simulink library "isi_correlator_lib"  (Simulink 7.4)
settings: Solver=ode45  SolverMode=SingleTasking  StartTime=0.0  StopTime=10.0  RelTol=1e-3
undefined symbols (not defined in the file or in its folder): latency
libraries: xbsIndex_r4 x341, isi_correlator_lib x33, casper_library x27, xps_library x7
(part 2 of 3)

== system isi_correlator_lib/scale ==
  din : Inport  OutDataType=sfix(16)  OutScaling=2^0
  scale : Inport  Port=2  OutDataType=sfix(16)  OutScaling=2^0
  Assert0 : xbsIndex_r4/Assert  assert_type=on  type_source=Explicitly  arith_type=Unsigned  n_bits=2 * data_bit_width  bin_pt=0  assert_rate=on  rate_source=Explicitly  period=1  output_port=on  block_type=assert
      settings: block_version=11.4
  Assert1 : xbsIndex_r4/Assert  assert_type=on  type_source=Explicitly  arith_type=Unsigned  n_bits=coef_bit_width  bin_pt=0  assert_rate=on  rate_source=Explicitly  period=1  output_port=on  block_type=assert
      settings: block_version=11.4
  Logical : xbsIndex_r4/Logical  logical_function=OR  inputs=2  en=off  latency=0  precision=Full  arith_type=Unsigned  n_bits=8  bin_pt=2  align_bp=on  dbl_ovrd=off  block_type=logical
      settings: xl_area=[0, 0, 0, 0, 0, 0, 0]
  Mult_imag : xbsIndex_r4/Mult  precision=Full  arith_type="Signed  (2's comp)"  n_bits=16  bin_pt=14  quantization=Truncate  overflow=Wrap  en=off  latency=3  dbl_ovrd=off  use_behavioral_HDL=off  opt=Speed  use_embedded=on  optimum_pipeline=off  pipeline=on  use_rpm=on  placement_style=Triangular  block_type=mult
      settings: infoedit=Hardware notes: To use the internal pipeline stage of the dedicated multiplier you must select 'Pipeline for maximum performance'.  block_version=10.1.3
  Mult_real : xbsIndex_r4/Mult  precision=Full  arith_type="Signed  (2's comp)"  n_bits=16  bin_pt=14  quantization=Truncate  overflow=Wrap  en=off  latency=3  dbl_ovrd=off  use_behavioral_HDL=off  opt=Speed  use_embedded=on  optimum_pipeline=off  pipeline=on  use_rpm=on  placement_style=Triangular  block_type=mult
      settings: infoedit=Hardware notes: To use the internal pipeline stage of the dedicated multiplier you must select 'Pipeline for maximum performance'.  block_version=10.1.3
  c_to_ri : casper_library/Misc/c_to_ri  SystemSampleTime=-1  n_bits=data_bit_width  bin_pt=data_bit_width - 1
      settings: AttributesFormatString=_ r/i
  ri_to_c : casper_library/Misc/ri_to_c  SystemSampleTime=-1
  saturate_imag : isi_correlator_lib/saturate  SystemSampleTime=-1  data_bit_width=data_bit_width  dout_bit_width=dout_bit_width
  saturate_real : isi_correlator_lib/saturate  SystemSampleTime=-1  data_bit_width=data_bit_width  dout_bit_width=dout_bit_width
  dout : Outport  OutDataType=sfix(16)  OutScaling=2^0
  clip : Outport  Port=2  OutDataType=sfix(16)  OutScaling=2^0
  wires:
  Assert1/1 -> Mult_real/2, Mult_imag/2
  c_to_ri/2 -> Mult_imag/1
  Logical/1 -> clip/1
  scale/1 -> Assert1/1
  c_to_ri/1 -> Mult_real/1
  ri_to_c/1 -> dout/1
  Mult_real/1 -> saturate_real/1
  Mult_imag/1 -> saturate_imag/1
  saturate_real/1 -> ri_to_c/1
  saturate_imag/1 -> ri_to_c/2
  saturate_real/2 -> Logical/1
  saturate_imag/2 -> Logical/2
  din/1 -> Assert0/1
  Assert0/1 -> c_to_ri/1

== system isi_correlator_lib/simple_bram_vacc ==
  new_acc : Inport  OutDataType=sfix(16)  OutScaling=2^0
  din : Inport  Port=2  OutDataType=sfix(16)  OutScaling=2^0
  Adder : xbsIndex_r4/AddSub  mode=Addition  use_carryin=off  use_carryout=off  en=off  latency=2  precision=User Defined  arith_type="Signed  (2's comp)"  n_bits=n_bits  bin_pt=bin_pt  quantization=Truncate  overflow=Wrap  dbl_ovrd=off  use_behavioral_HDL=off  hw_selection=Fabric  pipelined=on  use_rpm=on  block_type=addsub
      settings: xl_area=[0, 0, 0, 0, 0, 0, 0]  block_version=10.1.3
  Constant : xbsIndex_r4/Constant  arith_type=Signed (2's comp)  const=0  n_bits=n_bits  bin_pt=bin_pt  explicit_period=on  period=1  equ=P=C  opselect=C  inp2=PCIN>>17  opr=+  inp1=P  carry=CIN  dbl_ovrd=off  block_type=constant
  Mux : xbsIndex_r4/Mux  inputs=2  en=off  latency=0  precision=Full  arith_type="Signed  (2's comp)"  n_bits=8  bin_pt=2  quantization=Truncate  overflow=Wrap  dbl_ovrd=off  block_type=mux
      settings: xl_area=[0, 0, 0, 0, 0, 0, 0]
  delay_bram : Subsystem  mask(delay_bram){DelayLen=vec_len - 2, bram_latency=2}
      mask prompts: DelayLen "Delay By:"; bram_latency "BRAM Latency"
      mask help: A delay block that uses BRAM for its storage.
      mask init:
      | if (DelayLen <= bram_latency)
      | 	error('delay value must be greater than BRAM Latency');
      | end
      | BitWidth = max(ceil(log2(DelayLen)), 2);
      mask Help: eval('xlWeb(''http://casper.berkeley.edu/wiki/Delay_bram'')')
  pulse_ext : Subsystem  mask(pulse_ext){pulse_len=vec_len}
      mask prompts: pulse_len "Length of Pulse"
      mask help:
      | Extends a boolean signal to be high for the specified number of clocks after
      | the last high input.
      mask init:
      | bits = ceil(log2(pulse_len+1));
      mask Help: eval('xlWeb(''http://casper.berkeley.edu/wiki/Pulse_ext'')')
  dout : Outport  OutDataType=sfix(16)  OutScaling=2^0
  valid : Outport  Port=2  OutDataType=sfix(16)  OutScaling=2^0
  wires:
  Adder/1 -> delay_bram/1(In1)
  delay_bram/1(Out1) -> dout/1, Mux/2
  new_acc/1 -> pulse_ext/1(in)
  din/1 -> Adder/1
  pulse_ext/1(out) -> valid/1, Mux/1
  Mux/1 -> Adder/2
  Constant/1 -> Mux/3

== system isi_correlator_lib/sync_gen ==
  rst : Inport  OutDataType=sfix(16)  OutScaling=2^0
  AddSub : xbsIndex_r4/AddSub  mode=Subtraction  use_carryin=off  use_carryout=off  en=off  latency=2  precision=Full  arith_type=Unsigned  n_bits=16  bin_pt=14  quantization=Truncate  overflow=Wrap  dbl_ovrd=off  use_behavioral_HDL=off  hw_selection=Fabric  pipelined=off  use_rpm=on  block_type=addsub
      settings: block_version=10.1.3
  Delay : xbsIndex_r4/Delay  en=off  latency=3  dbl_ovrd=off  reg_retiming=on  block_type=delay
      settings: block_version=11.3
  Logical1 : xbsIndex_r4/Logical  logical_function=OR  inputs=2  en=off  latency=0  precision=Full  arith_type=Unsigned  n_bits=16  bin_pt=0  align_bp=on  dbl_ovrd=off  block_type=logical
  Relational : xbsIndex_r4/Relational  mode=a>=b  en=off  latency=1  dbl_ovrd=off  block_type=relational
      settings: block_version=10.1.3
  counter : xbsIndex_r4/Counter  cnt_type=Free Running  cnt_to=Inf  operation=Up  start_count=0  cnt_by_val=1  arith_type=Unsigned  n_bits=32  bin_pt=0  load_pin=off  rst=on  en=off  explicit_period=on  period=1  dbl_ovrd=off  use_behavioral_HDL=off  implementation=Fabric  use_rpm=off  block_type=counter
  default_period : Constant  Value=1024  OutDataType=sfix(16)  OutScaling=2^0  SampleTime=1
  period : xps_library/software register  Tag=xps:sw_reg  SystemSampleTime=-1  io_dir=From Processor  arith_type=Unsigned  bitwidth=32  bin_pt=0  sample_period=1  gw_name=isi_correlator_lib_sync_gen_period_user_data_out
  period_offset : xbsIndex_r4/Constant  arith_type=Unsigned  const=3  n_bits=32  bin_pt=0  explicit_period=on  period=1  equ=P=C  opselect=C  inp2=PCIN>>17  opr=+  inp1=P  carry=CIN  dbl_ovrd=off  block_type=constant
      settings: block_version=10.1.1
  posedge : casper_library/Misc/posedge  Tag=Rising Edge Detector  SystemSampleTime=-1
  sync : Outport  OutDataType=sfix(16)  OutScaling=2^0
  wires:
  rst/1 -> Logical1/2
  Relational/1 -> Logical1/1
  posedge/1 -> sync/1
  Logical1/1 -> counter/1, posedge/1
  counter/1 -> Relational/1
  AddSub/1 -> Relational/2
  period_offset/1 -> AddSub/2
  default_period/1 -> period/1
  period/1 -> Delay/1
  Delay/1 -> AddSub/1

== system isi_correlator_lib/synced_cntr ==
  sync : Inport
  Constant : xbsIndex_r4/Constant  arith_type=Unsigned  const=0  n_bits=nextpow2(period)  bin_pt=0  explicit_period=on  period=1  equ=P=C  opselect=C  inp2=PCIN>>17  opr=+  inp1=P  carry=CIN  dbl_ovrd=off  block_type=constant
      settings: block_version=11.4
  Constant3 : xbsIndex_r4/Constant  arith_type=Unsigned  const=period - 1  n_bits=nextpow2(period)  bin_pt=0  explicit_period=on  period=1  equ=P=C  opselect=C  inp2=PCIN>>17  opr=+  inp1=P  carry=CIN  dbl_ovrd=off  block_type=constant
      settings: block_version=11.4
  Counter : xbsIndex_r4/Counter  cnt_type=Free Running  cnt_to=Inf  operation=Up  start_count=0  cnt_by_val=1  arith_type=Unsigned  n_bits=nextpow2(period)  bin_pt=0  load_pin=on  rst=off  en=off  explicit_period=on  period=1  dbl_ovrd=off  use_behavioral_HDL=off  implementation=Fabric  use_rpm=off  block_type=counter
  Logical2 : xbsIndex_r4/Logical  logical_function=OR  inputs=2  en=off  latency=0  precision=Full  arith_type=Unsigned  n_bits=16  bin_pt=0  align_bp=on  dbl_ovrd=off  block_type=logical
      settings: block_version=11.3
  Relational2 : xbsIndex_r4/Relational  mode=a=b  en=off  latency=0  dbl_ovrd=off  block_type=relational
  cnt : Outport
  wires:
  Constant/1 -> Counter/2
  sync/1 -> Logical2/2
  Logical2/1 -> Counter/1
  Counter/1 -> cnt/1, Relational2/2
  Constant3/1 -> Relational2/1
  Relational2/1 -> Logical2/1

== system isi_correlator_lib/trig_cntr ==
  trig : Inport
  Counter : xbsIndex_r4/Counter  cnt_type=Free Running  cnt_to=Inf  operation=Up  start_count=0  cnt_by_val=1  arith_type=Unsigned  n_bits=bitwidth + 1  bin_pt=0  load_pin=off  rst=on  en=on  explicit_period=on  period=1  dbl_ovrd=off  use_behavioral_HDL=off  implementation=Fabric  use_rpm=off  block_type=counter
  Inverter : xbsIndex_r4/Inverter  en=off  latency=0  dbl_ovrd=off  block_type=inv
      settings: block_version=11.3
  Inverter1 : xbsIndex_r4/Inverter  en=off  latency=0  dbl_ovrd=off  block_type=inv
      settings: block_version=11.3
  Logical : xbsIndex_r4/Logical  logical_function=AND  inputs=2  en=off  latency=latency  precision=Full  arith_type=Unsigned  n_bits=16  bin_pt=0  align_bp=on  dbl_ovrd=off  block_type=logical
      settings: block_version=11.3
  address : xbsIndex_r4/Slice  nbits=bitwidth  boolean_output=off  mode=Lower Bit Location + Width  bit1=0  base1=MSB of Input  bit0=0  base0=LSB of Input  dbl_ovrd=off  block_type=slice
      settings: block_version=10.1.1
  cntr_delay0 : xbsIndex_r4/Delay  en=off  latency=latency  dbl_ovrd=off  reg_retiming=on  block_type=delay
      settings: block_version=11.3
  overflow : xbsIndex_r4/Slice  nbits=1  boolean_output=on  mode=Upper Bit Location + Width  bit1=0  base1=MSB of Input  bit0=0  base0=LSB of Input  dbl_ovrd=off  block_type=slice
      settings: block_version=10.1.1
  addr : Outport
  we : Outport  Port=2
  wires:
  Counter/1 -> overflow/1, address/1
  trig/1 -> Counter/1, Inverter1/1
  address/1 -> cntr_delay0/1
  overflow/1 -> Inverter/1
  Inverter/1 -> Counter/2, Logical/1
  Inverter1/1 -> Logical/2
  Logical/1 -> we/1
  cntr_delay0/1 -> addr/1

== system isi_correlator_lib/tvg ==
  sync : Inport
  Constant : xbsIndex_r4/Constant  arith_type=Unsigned  const=0  n_bits=32  bin_pt=0  explicit_period=on  period=1  equ=P=C  opselect=C  inp2=PCIN>>17  opr=+  inp1=P  carry=CIN  dbl_ovrd=off  block_type=constant
  Constant1 : xbsIndex_r4/Constant  arith_type=Boolean  const=0  n_bits=32  bin_pt=0  explicit_period=on  period=1  equ=P=C  opselect=C  inp2=PCIN>>17  opr=+  inp1=P  carry=CIN  dbl_ovrd=off  block_type=constant
  bram : xps_library/Shared BRAM  Tag=xps:bram  SystemSampleTime=-1  arith_type="Signed  (2's comp)"  addr_width=nextpow2(length)  data_width=32  data_bin_pt=0  init_vals=[1:2^nextpow2(length)]  sample_rate=1
  delay3 : xbsIndex_r4/Delay  en=off  latency=1  dbl_ovrd=off  reg_retiming=off  block_type=delay
  synced_cntr : isi_correlator_lib/synced_cntr  SystemSampleTime=-1  period=length
  sync_out : Outport
  dout : Outport  Port=2
  wires:
  delay3/1 -> sync_out/1
  bram/1 -> dout/1
  synced_cntr/1 -> bram/1
  sync/1 -> delay3/1, synced_cntr/1
  Constant/1 -> bram/2
  Constant1/1 -> bram/3

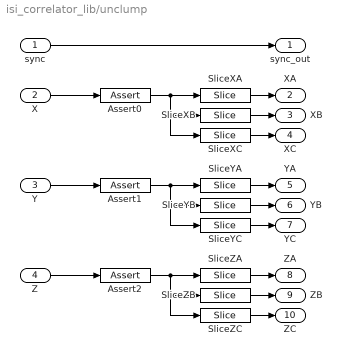
== system isi_correlator_lib/unclump ==
  sync : Inport
  X : Inport  Port=2
  Y : Inport  Port=3
  Z : Inport  Port=4
  Assert0 : xbsIndex_r4/Assert  assert_type=on  type_source=Explicitly  arith_type=Unsigned  n_bits=24  bin_pt=0  assert_rate=on  rate_source=Explicitly  period=1  output_port=on  block_type=assert
      settings: block_version=11.4
  Assert1 : xbsIndex_r4/Assert  assert_type=on  type_source=Explicitly  arith_type=Unsigned  n_bits=24  bin_pt=0  assert_rate=on  rate_source=Explicitly  period=1  output_port=on  block_type=assert
      settings: block_version=11.4
  Assert2 : xbsIndex_r4/Assert  assert_type=on  type_source=Explicitly  arith_type=Unsigned  n_bits=24  bin_pt=0  assert_rate=on  rate_source=Explicitly  period=1  output_port=on  block_type=assert
      settings: block_version=11.4
  SliceXA : xbsIndex_r4/Slice  nbits=8  boolean_output=off  mode=Lower Bit Location + Width  bit1=0  base1=MSB of Input  bit0=16  base0=LSB of Input  dbl_ovrd=off  block_type=slice
      settings: block_version=10.1.1
  SliceXB : xbsIndex_r4/Slice  nbits=8  boolean_output=off  mode=Lower Bit Location + Width  bit1=0  base1=MSB of Input  bit0=8  base0=LSB of Input  dbl_ovrd=off  block_type=slice
      settings: block_version=10.1.1
  SliceXC : xbsIndex_r4/Slice  nbits=8  boolean_output=off  mode=Lower Bit Location + Width  bit1=0  base1=MSB of Input  bit0=0  base0=LSB of Input  dbl_ovrd=off  block_type=slice
      settings: block_version=10.1.1
  SliceYA : xbsIndex_r4/Slice  nbits=8  boolean_output=off  mode=Lower Bit Location + Width  bit1=0  base1=MSB of Input  bit0=16  base0=LSB of Input  dbl_ovrd=off  block_type=slice
      settings: block_version=10.1.1
  SliceYB : xbsIndex_r4/Slice  nbits=8  boolean_output=off  mode=Lower Bit Location + Width  bit1=0  base1=MSB of Input  bit0=8  base0=LSB of Input  dbl_ovrd=off  block_type=slice
      settings: block_version=10.1.1
  SliceYC : xbsIndex_r4/Slice  nbits=8  boolean_output=off  mode=Lower Bit Location + Width  bit1=0  base1=MSB of Input  bit0=0  base0=LSB of Input  dbl_ovrd=off  block_type=slice
      settings: block_version=10.1.1
  SliceZA : xbsIndex_r4/Slice  nbits=8  boolean_output=off  mode=Lower Bit Location + Width  bit1=0  base1=MSB of Input  bit0=16  base0=LSB of Input  dbl_ovrd=off  block_type=slice
      settings: block_version=10.1.1
  SliceZB : xbsIndex_r4/Slice  nbits=8  boolean_output=off  mode=Lower Bit Location + Width  bit1=0  base1=MSB of Input  bit0=8  base0=LSB of Input  dbl_ovrd=off  block_type=slice
      settings: block_version=10.1.1
  SliceZC : xbsIndex_r4/Slice  nbits=8  boolean_output=off  mode=Lower Bit Location + Width  bit1=0  base1=MSB of Input  bit0=0  base0=LSB of Input  dbl_ovrd=off  block_type=slice
      settings: block_version=10.1.1
  sync_out : Outport
  XA : Outport  Port=2
  XB : Outport  Port=3
  XC : Outport  Port=4
  YA : Outport  Port=5
  YB : Outport  Port=6
  YC : Outport  Port=7
  ZA : Outport  Port=8
  ZB : Outport  Port=9
  ZC : Outport  Port=10
  wires:
  SliceZC/1 -> ZC/1
  SliceZB/1 -> ZB/1
  SliceZA/1 -> ZA/1
  SliceYC/1 -> YC/1
  SliceYB/1 -> YB/1
  SliceYA/1 -> YA/1
  SliceXC/1 -> XC/1
  SliceXB/1 -> XB/1
  SliceXA/1 -> XA/1
  Assert2/1 -> SliceZB/1, SliceZC/1, SliceZA/1
  Assert1/1 -> SliceYB/1, SliceYC/1, SliceYA/1
  Assert0/1 -> SliceXB/1, SliceXC/1, SliceXA/1
  Z/1 -> Assert2/1
  Y/1 -> Assert1/1
  X/1 -> Assert0/1
  sync/1 -> sync_out/1

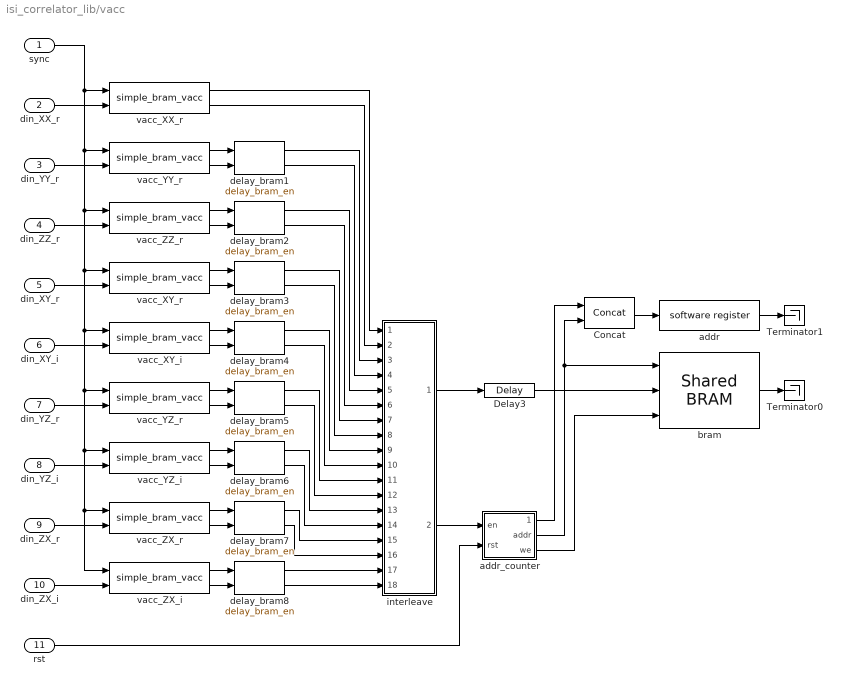
== system isi_correlator_lib/vacc ==
  sync : Inport
  din_XX_r : Inport  Port=2
  din_YY_r : Inport  Port=3
  din_ZZ_r : Inport  Port=4
  din_XY_r : Inport  Port=5
  din_XY_i : Inport  Port=6
  din_YZ_r : Inport  Port=7
  din_YZ_i : Inport  Port=8
  din_ZX_r : Inport  Port=9
  din_ZX_i : Inport  Port=10
  rst : Inport  Port=11
  Concat : xbsIndex_r4/Concat  num_inputs=2  dbl_ovrd=off  block_type=concat
  Delay3 : xbsIndex_r4/Delay  en=off  latency=1  dbl_ovrd=off  reg_retiming=off  block_type=delay
      settings: xl_area=[0, 0, 0, 0, 0, 0, 0]  block_version=9.1.01
  Terminator0 : Terminator
  Terminator1 : Terminator
  addr : xps_library/software register  Tag=xps:sw_reg  SystemSampleTime=-1  io_dir=To Processor  arith_type=Unsigned  bitwidth=32  bin_pt=0  sample_period=1  gw_name=isi_correlator_lib_vacc_addr_user_data_in
  addr_counter : Subsystem
  bram : xps_library/Shared BRAM  Tag=xps:bram  SystemSampleTime=-1  arith_type="Signed  (2's comp)"  addr_width=10  data_width=32  data_bin_pt=out_bin_point  init_vals=0  sample_rate=1
  delay_bram1 : isi_correlator_lib/delay_bram_en  SystemSampleTime=-1  DelayLen=1 * vector_length  bram_latency=2
  delay_bram2 : isi_correlator_lib/delay_bram_en  SystemSampleTime=-1  DelayLen=2 * vector_length  bram_latency=2
  delay_bram3 : isi_correlator_lib/delay_bram_en  SystemSampleTime=-1  DelayLen=3 * vector_length  bram_latency=2
  delay_bram4 : isi_correlator_lib/delay_bram_en  SystemSampleTime=-1  DelayLen=4 * vector_length  bram_latency=2
  delay_bram5 : isi_correlator_lib/delay_bram_en  SystemSampleTime=-1  DelayLen=5*vector_length  bram_latency=2
  delay_bram6 : isi_correlator_lib/delay_bram_en  SystemSampleTime=-1  DelayLen=6 * vector_length  bram_latency=2
  delay_bram7 : isi_correlator_lib/delay_bram_en  SystemSampleTime=-1  DelayLen=7 * vector_length  bram_latency=2
  delay_bram8 : isi_correlator_lib/delay_bram_en  SystemSampleTime=-1  DelayLen=8 * vector_length  bram_latency=2
  interleave : Subsystem  mask{bit_width=out_bit_width, bin_point=out_bin_point, logic_latency=1, fanin_latency=fanin_latency}
      mask prompts: bit_width "Bit width:"; bin_point "Binary point:"; logic_latency "Logic latency:"; fanin_latency "Fanin latency:"
  vacc_XX_r : casper_library/Accumulators/simple_bram_vacc  SystemSampleTime=-1  vec_len=vector_length  arith_type=Signed  n_bits=out_bit_width  bin_pt=out_bin_point
  vacc_XY_i : casper_library/Accumulators/simple_bram_vacc  SystemSampleTime=-1  vec_len=vector_length  arith_type=Signed  n_bits=out_bit_width  bin_pt=out_bin_point
  vacc_XY_r : casper_library/Accumulators/simple_bram_vacc  SystemSampleTime=-1  vec_len=vector_length  arith_type=Signed  n_bits=out_bit_width  bin_pt=out_bin_point
  vacc_YY_r : casper_library/Accumulators/simple_bram_vacc  SystemSampleTime=-1  vec_len=vector_length  arith_type=Signed  n_bits=out_bit_width  bin_pt=out_bin_point
  vacc_YZ_i : casper_library/Accumulators/simple_bram_vacc  SystemSampleTime=-1  vec_len=vector_length  arith_type=Signed  n_bits=out_bit_width  bin_pt=out_bin_point
  vacc_YZ_r : casper_library/Accumulators/simple_bram_vacc  SystemSampleTime=-1  vec_len=vector_length  arith_type=Signed  n_bits=out_bit_width  bin_pt=out_bin_point
  vacc_ZX_i : casper_library/Accumulators/simple_bram_vacc  SystemSampleTime=-1  vec_len=vector_length  arith_type=Signed  n_bits=out_bit_width  bin_pt=out_bin_point
  vacc_ZX_r : casper_library/Accumulators/simple_bram_vacc  SystemSampleTime=-1  vec_len=vector_length  arith_type=Signed  n_bits=out_bit_width  bin_pt=out_bin_point
  vacc_ZZ_r : casper_library/Accumulators/simple_bram_vacc  SystemSampleTime=-1  vec_len=vector_length  arith_type=Signed  n_bits=out_bit_width  bin_pt=out_bin_point
  wires:
  Delay3/1 -> bram/2
  bram/1 -> Terminator0/1
  din_ZX_i/1 -> vacc_ZX_i/2
  din_ZX_r/1 -> vacc_ZX_r/2
  din_YZ_i/1 -> vacc_YZ_i/2
  din_YZ_r/1 -> vacc_YZ_r/2
  din_XY_i/1 -> vacc_XY_i/2
  din_XY_r/1 -> vacc_XY_r/2
  din_ZZ_r/1 -> vacc_ZZ_r/2
  din_YY_r/1 -> vacc_YY_r/2
  din_XX_r/1 -> vacc_XX_r/2
  sync/1 -> vacc_XX_r/1, vacc_ZZ_r/1, vacc_XY_r/1, vacc_XY_i/1, vacc_YZ_r/1, vacc_YZ_i/1, vacc_ZX_r/1, vacc_ZX_i/1, vacc_YY_r/1
  vacc_ZZ_r/1 -> delay_bram2/1
  vacc_ZZ_r/2 -> delay_bram2/2
  vacc_XY_r/1 -> delay_bram3/1
  vacc_XY_r/2 -> delay_bram3/2
  vacc_XY_i/1 -> delay_bram4/1
  vacc_XY_i/2 -> delay_bram4/2
  vacc_YZ_r/1 -> delay_bram5/1
  vacc_YZ_r/2 -> delay_bram5/2
  vacc_YY_r/1 -> delay_bram1/1
  vacc_YY_r/2 -> delay_bram1/2
  vacc_ZX_i/1 -> delay_bram8/1
  vacc_ZX_i/2 -> delay_bram8/2
  vacc_ZX_r/1 -> delay_bram7/1
  vacc_ZX_r/2 -> delay_bram7/2
  vacc_YZ_i/1 -> delay_bram6/1
  vacc_YZ_i/2 -> delay_bram6/2
  vacc_XX_r/1 -> interleave/1(data0)
  vacc_XX_r/2 -> interleave/2(valid0)
  delay_bram1/1 -> interleave/3(data1)
  delay_bram1/2 -> interleave/4(valid1)
  delay_bram2/1 -> interleave/5(data2)
  delay_bram2/2 -> interleave/6(valid2)
  delay_bram3/1 -> interleave/7(data3)
  delay_bram3/2 -> interleave/8(valid3)
  rst/1 -> addr_counter/2(rst)
  delay_bram8/1 -> interleave/17(data8)
  delay_bram8/2 -> interleave/18(valid8)
  delay_bram4/1 -> interleave/9(data4)
  delay_bram4/2 -> interleave/10(valid4)
  delay_bram5/1 -> interleave/11(data5)
  delay_bram5/2 -> interleave/12(valid5)
  delay_bram6/1 -> interleave/13(data6)
  delay_bram6/2 -> interleave/14(valid6)
  delay_bram7/1 -> interleave/15(data7)
  delay_bram7/2 -> interleave/16(valid7)
  interleave/2(valid) -> addr_counter/1(en)
  interleave/1(data) -> Delay3/1
  addr_counter/3(we) -> bram/3
  addr/1 -> Terminator1/1
  Concat/1 -> addr/1
  addr_counter/2(addr) -> bram/1, Concat/2
  addr_counter/1(pkt_id) -> Concat/1

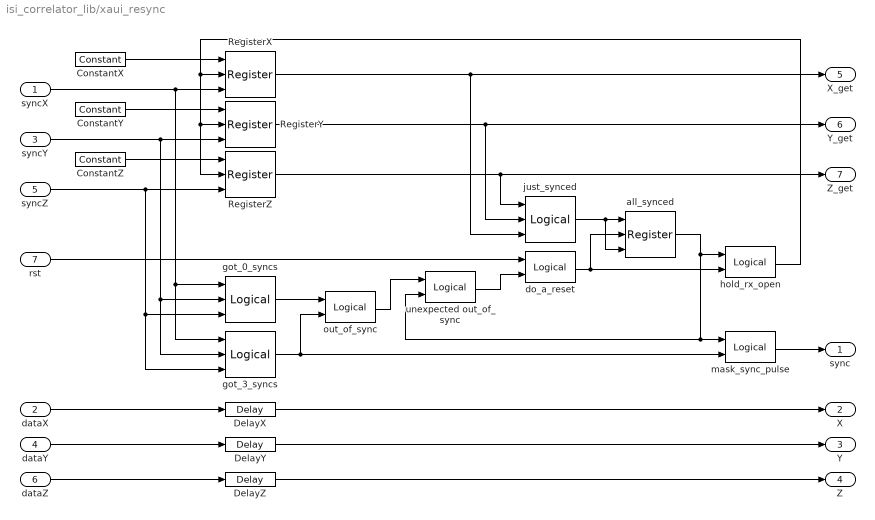
== system isi_correlator_lib/xaui_resync ==
  syncX : Inport  OutDataType=sfix(16)  OutScaling=2^0
  dataX : Inport  Port=2  OutDataType=sfix(16)  OutScaling=2^0
  syncY : Inport  Port=3  OutDataType=sfix(16)  OutScaling=2^0
  dataY : Inport  Port=4  OutDataType=sfix(16)  OutScaling=2^0
  syncZ : Inport  Port=5  OutDataType=sfix(16)  OutScaling=2^0
  dataZ : Inport  Port=6  OutDataType=sfix(16)  OutScaling=2^0
  rst : Inport  Port=7  OutDataType=sfix(16)  OutScaling=2^0
  ConstantX : xbsIndex_r4/Constant  arith_type=Boolean  const=0  n_bits=1  bin_pt=0  explicit_period=on  period=1  equ=P=C  opselect=C  inp2=PCIN>>17  opr=+  inp1=P  carry=CIN  dbl_ovrd=off  block_type=constant
      settings: block_version=10.1.1
  ConstantY : xbsIndex_r4/Constant  arith_type=Boolean  const=0  n_bits=1  bin_pt=0  explicit_period=on  period=1  equ=P=C  opselect=C  inp2=PCIN>>17  opr=+  inp1=P  carry=CIN  dbl_ovrd=off  block_type=constant
      settings: block_version=10.1.1
  ConstantZ : xbsIndex_r4/Constant  arith_type=Boolean  const=0  n_bits=1  bin_pt=0  explicit_period=on  period=1  equ=P=C  opselect=C  inp2=PCIN>>17  opr=+  inp1=P  carry=CIN  dbl_ovrd=off  block_type=constant
      settings: block_version=10.1.1
  DelayX : xbsIndex_r4/Delay  en=off  latency=1  dbl_ovrd=off  reg_retiming=on  block_type=delay
  DelayY : xbsIndex_r4/Delay  en=off  latency=1  dbl_ovrd=off  reg_retiming=on  block_type=delay
  DelayZ : xbsIndex_r4/Delay  en=off  latency=1  dbl_ovrd=off  reg_retiming=on  block_type=delay
  RegisterX : xbsIndex_r4/Register  init=1  rst=on  en=on  dbl_ovrd=off  block_type=register
      settings: block_version=11.4
  RegisterY : xbsIndex_r4/Register  init=1  rst=on  en=on  dbl_ovrd=off  block_type=register
      settings: block_version=11.4
  RegisterZ : xbsIndex_r4/Register  init=1  rst=on  en=on  dbl_ovrd=off  block_type=register
      settings: block_version=11.4
  all_synced : xbsIndex_r4/Register  init=0  rst=on  en=on  dbl_ovrd=off  block_type=register
      settings: block_version=11.4
  do_a_reset : xbsIndex_r4/Logical  logical_function=OR  inputs=2  en=off  latency=1  precision=Full  arith_type=Unsigned  n_bits=16  bin_pt=0  align_bp=on  dbl_ovrd=off  block_type=logical
      settings: block_version=11.4
  got_0_syncs : xbsIndex_r4/Logical  logical_function=NOR  inputs=3  en=off  latency=1  precision=Full  arith_type=Unsigned  n_bits=16  bin_pt=0  align_bp=on  dbl_ovrd=off  block_type=logical
      settings: block_version=11.4
  got_3_syncs : xbsIndex_r4/Logical  logical_function=AND  inputs=3  en=off  latency=1  precision=Full  arith_type=Unsigned  n_bits=16  bin_pt=0  align_bp=on  dbl_ovrd=off  block_type=logical
      settings: block_version=11.4
  hold_rx_open : xbsIndex_r4/Logical  logical_function=OR  inputs=2  en=off  latency=0  precision=Full  arith_type=Unsigned  n_bits=16  bin_pt=0  align_bp=on  dbl_ovrd=off  block_type=logical
      settings: block_version=11.4
  just_synced : xbsIndex_r4/Logical  logical_function=NOR  inputs=3  en=off  latency=depth - 2  precision=Full  arith_type=Unsigned  n_bits=16  bin_pt=0  align_bp=on  dbl_ovrd=off  block_type=logical
      settings: block_version=11.4
  mask_sync_pulse : xbsIndex_r4/Logical  logical_function=AND  inputs=2  en=off  latency=0  precision=Full  arith_type=Unsigned  n_bits=16  bin_pt=0  align_bp=on  dbl_ovrd=off  block_type=logical
      settings: block_version=11.4
  out_of_sync : xbsIndex_r4/Logical  logical_function=NOR  inputs=2  en=off  latency=0  precision=Full  arith_type=Unsigned  n_bits=16  bin_pt=0  align_bp=on  dbl_ovrd=off  block_type=logical
      settings: block_version=11.4
  unexpected out_of_sync : xbsIndex_r4/Logical  logical_function=AND  inputs=2  en=off  latency=0  precision=Full  arith_type=Unsigned  n_bits=16  bin_pt=0  align_bp=on  dbl_ovrd=off  block_type=logical
      settings: block_version=11.4
  sync : Outport  OutDataType=sfix(16)  OutScaling=2^0
  X : Outport  Port=2  OutDataType=sfix(16)  OutScaling=2^0
  Y : Outport  Port=3  OutDataType=sfix(16)  OutScaling=2^0
  Z : Outport  Port=4  OutDataType=sfix(16)  OutScaling=2^0
  X_get : Outport  Port=5  OutDataType=sfix(16)  OutScaling=2^0
  Y_get : Outport  Port=6  OutDataType=sfix(16)  OutScaling=2^0
  Z_get : Outport  Port=7  OutDataType=sfix(16)  OutScaling=2^0
  wires:
  hold_rx_open/1 -> RegisterY/2, RegisterZ/2, RegisterX/2
  unexpected out_of_sync/1 -> do_a_reset/2
  out_of_sync/1 -> unexpected out_of_sync/1
  got_0_syncs/1 -> out_of_sync/1
  got_3_syncs/1 -> out_of_sync/2, mask_sync_pulse/2
  rst/1 -> do_a_reset/1
  do_a_reset/1 -> all_synced/2, hold_rx_open/2
  dataX/1 -> DelayX/1
  DelayZ/1 -> Z/1
  DelayY/1 -> Y/1
  DelayX/1 -> X/1
  mask_sync_pulse/1 -> sync/1
  all_synced/1 -> unexpected out_of_sync/2, mask_sync_pulse/1, hold_rx_open/1
  just_synced/1 -> all_synced/3, all_synced/1
  RegisterZ/1 -> just_synced/1, Z_get/1
  RegisterX/1 -> just_synced/3, X_get/1
  RegisterY/1 -> just_synced/2, Y_get/1
  dataZ/1 -> DelayZ/1
  dataY/1 -> DelayY/1
  syncZ/1 -> got_3_syncs/3, got_0_syncs/3, RegisterZ/3
  syncY/1 -> got_3_syncs/2, got_0_syncs/2, RegisterY/3
  syncX/1 -> got_3_syncs/1, got_0_syncs/1, RegisterX/3
  ConstantZ/1 -> RegisterZ/1
  ConstantY/1 -> RegisterY/1
  ConstantX/1 -> RegisterX/1

== system isi_correlator_lib/packed_bram/addr_counter ==
  en : Inport
  rst : Inport  Port=2
  Constant3 : xbsIndex_r4/Constant  arith_type=Unsigned  const=num_words - 1  n_bits=nextpow2(num_words)  bin_pt=0  explicit_period=on  period=1  equ=P=C  opselect=C  inp2=PCIN>>17  opr=+  inp1=P  carry=CIN  dbl_ovrd=off  block_type=constant
      settings: block_version=11.4
  Constant4 : xbsIndex_r4/Constant  arith_type=Unsigned  const=0  n_bits=nextpow2(num_words)  bin_pt=0  explicit_period=on  period=1  equ=P=C  opselect=C  inp2=PCIN>>17  opr=+  inp1=P  carry=CIN  dbl_ovrd=off  block_type=constant
      settings: block_version=11.4
  Inverter : xbsIndex_r4/Inverter  en=off  latency=0  dbl_ovrd=off  block_type=inv
      settings: block_version=11.3
  Logical1 : xbsIndex_r4/Logical  logical_function=AND  inputs=2  en=off  latency=0  precision=Full  arith_type=Unsigned  n_bits=16  bin_pt=0  align_bp=on  dbl_ovrd=off  block_type=logical
      settings: block_version=11.3
  Logical2 : xbsIndex_r4/Logical  logical_function=OR  inputs=2  en=off  latency=0  precision=Full  arith_type=Unsigned  n_bits=16  bin_pt=0  align_bp=on  dbl_ovrd=off  block_type=logical
      settings: block_version=11.3
  Logical3 : xbsIndex_r4/Logical  logical_function=OR  inputs=2  en=off  latency=0  precision=Full  arith_type=Unsigned  n_bits=16  bin_pt=0  align_bp=on  dbl_ovrd=off  block_type=logical
      settings: block_version=11.3
  Relational2 : xbsIndex_r4/Relational  mode=a=b  en=off  latency=0  dbl_ovrd=off  block_type=relational
  bram_addr : xbsIndex_r4/Counter  cnt_type=Free Running  cnt_to=Inf  operation=Up  start_count=0  cnt_by_val=1  arith_type=Unsigned  n_bits=nextpow2(num_words)  bin_pt=0  load_pin=on  rst=off  en=on  explicit_period=on  period=1  dbl_ovrd=off  use_behavioral_HDL=off  implementation=Fabric  use_rpm=off  block_type=counter
  packet_id : xbsIndex_r4/Counter  cnt_type=Free Running  cnt_to=Inf  operation=Up  start_count=0  cnt_by_val=1  arith_type=Unsigned  n_bits=32  bin_pt=0  load_pin=off  rst=on  en=on  explicit_period=on  period=1  dbl_ovrd=off  use_behavioral_HDL=off  implementation=Fabric  use_rpm=off  block_type=counter
  rst_filter : Subsystem
  pkt_id : Outport
  addr : Outport  Port=2
  we : Outport  Port=3
  wires:
  rst_filter/1(e) -> Logical1/1, Logical3/2
  rst_filter/2(r) -> Logical2/2, packet_id/1, Inverter/1
  Inverter/1 -> Logical1/2
  Relational2/1 -> packet_id/2, Logical2/1
  Logical1/1 -> we/1
  Constant3/1 -> Relational2/1
  bram_addr/1 -> Relational2/2, addr/1
  rst/1 -> rst_filter/2(rst)
  en/1 -> rst_filter/1(en)
  Logical3/1 -> bram_addr/3
  Constant4/1 -> bram_addr/2
  Logical2/1 -> Logical3/1, bram_addr/1
  packet_id/1 -> pkt_id/1

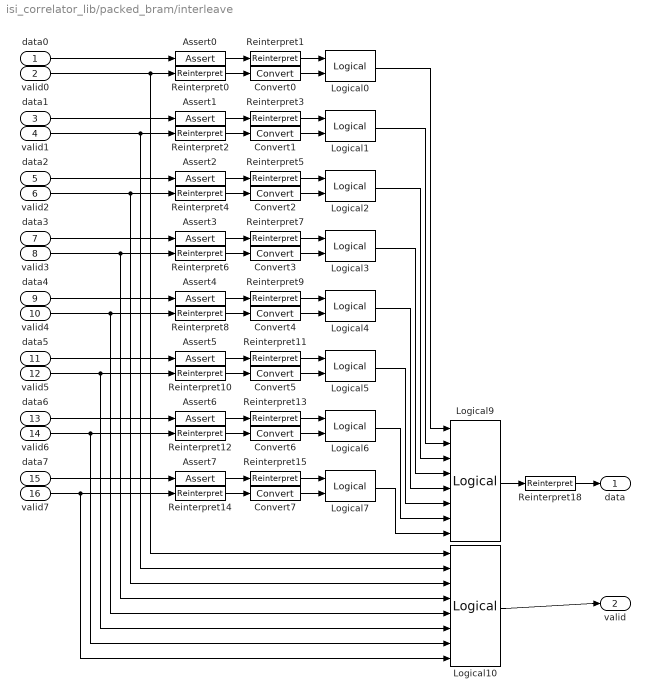
== system isi_correlator_lib/packed_bram/interleave ==
  data0 : Inport
  valid0 : Inport  Port=2
  data1 : Inport  Port=3
  valid1 : Inport  Port=4
  data2 : Inport  Port=5
  valid2 : Inport  Port=6
  data3 : Inport  Port=7
  valid3 : Inport  Port=8
  data4 : Inport  Port=9
  valid4 : Inport  Port=10
  data5 : Inport  Port=11
  valid5 : Inport  Port=12
  data6 : Inport  Port=13
  valid6 : Inport  Port=14
  data7 : Inport  Port=15
  valid7 : Inport  Port=16
  Assert{0..7} (8 alike) : xbsIndex_r4/Assert  assert_type=off  type_source=Explicitly  arith_type="Signed  (2's comp)"  n_bits=bit_width  bin_pt=bin_point  assert_rate=on  rate_source=Explicitly  period=1  output_port=on  block_type=assert
      settings: block_version=11.4
  Convert{0..7} (8 alike) : xbsIndex_r4/Convert  arith_type="Signed  (2's comp)"  n_bits=bit_width  bin_pt=0  quantization=Truncate  overflow=Wrap  latency=0  dbl_ovrd=off  pipeline=off  block_type=convert
      settings: block_version=11.4
  Logical{0..7} (8 alike) : xbsIndex_r4/Logical  logical_function=AND  inputs=2  en=off  latency=logic_latency  precision=Full  arith_type=Unsigned  n_bits=16  bin_pt=0  align_bp=on  dbl_ovrd=off  block_type=logical
      settings: block_version=11.3
  Logical10 : xbsIndex_r4/Logical  logical_function=OR  inputs=8  en=off  latency=logic_latency + fanin_latency  precision=Full  arith_type=Unsigned  n_bits=16  bin_pt=0  align_bp=on  dbl_ovrd=off  block_type=logical
      settings: block_version=11.3
  Logical9 : xbsIndex_r4/Logical  logical_function=OR  inputs=8  en=off  latency=fanin_latency  precision=Full  arith_type=Unsigned  n_bits=16  bin_pt=0  align_bp=on  dbl_ovrd=off  block_type=logical
      settings: block_version=11.3
  Reinterpret{0,2,4,6,8,10,12,14} (8 alike) : xbsIndex_r4/Reinterpret  force_arith_type=on  arith_type="Signed  (2's comp)"  force_bin_pt=on  bin_pt=0  block_type=reinterpret
      settings: infoedit="Changes signal type without altering the binary representation.   You can changed the signal between signed and unsigned, and relocate the binary point.<br><br>Hardware notes: In hardware this block costs nothing.<br><br>Example:  Suppose the input is 6 bits wide, signed, with 2 fractional bits, and the output is forced to unsigned with 0 fractional bits.  Then an input of -2.0 (1110.00 in binary 2's complement) becomes an output of 56 (111000 in binary)."
  Reinterpret{1,3,5,7,9,11,13,15} (8 alike) : xbsIndex_r4/Reinterpret  force_arith_type=on  arith_type=Unsigned  force_bin_pt=on  bin_pt=0  block_type=reinterpret
      settings: infoedit="Changes signal type without altering the binary representation.   You can changed the signal between signed and unsigned, and relocate the binary point.<br><br>Hardware notes: In hardware this block costs nothing.<br><br>Example:  Suppose the input is 6 bits wide, signed, with 2 fractional bits, and the output is forced to unsigned with 0 fractional bits.  Then an input of -2.0 (1110.00 in binary 2's complement) becomes an output of 56 (111000 in binary)."
  Reinterpret18 : xbsIndex_r4/Reinterpret  force_arith_type=on  arith_type="Signed  (2's comp)"  force_bin_pt=off  bin_pt=bin_point  block_type=reinterpret
      settings: infoedit="Changes signal type without altering the binary representation.   You can changed the signal between signed and unsigned, and relocate the binary point.<br><br>Hardware notes: In hardware this block costs nothing.<br><br>Example:  Suppose the input is 6 bits wide, signed, with 2 fractional bits, and the output is forced to unsigned with 0 fractional bits.  Then an input of -2.0 (1110.00 in binary 2's complement) becomes an output of 56 (111000 in binary)."
  data : Outport
  valid : Outport  Port=2
  wires:
  Logical7/1 -> Logical9/8
  Logical6/1 -> Logical9/7
  Logical5/1 -> Logical9/6
  Logical4/1 -> Logical9/5
  Logical3/1 -> Logical9/4
  Logical2/1 -> Logical9/3
  Logical1/1 -> Logical9/2
  Logical0/1 -> Logical9/1
  Logical10/1 -> valid/1
  Reinterpret18/1 -> data/1
  Logical9/1 -> Reinterpret18/1
  valid7/1 -> Logical10/8, Reinterpret14/1
  data7/1 -> Assert7/1
  valid6/1 -> Logical10/7, Reinterpret12/1
  data6/1 -> Assert6/1
  valid5/1 -> Logical10/6, Reinterpret10/1
  data5/1 -> Assert5/1
  valid4/1 -> Logical10/5, Reinterpret8/1
  data4/1 -> Assert4/1
  valid3/1 -> Logical10/4, Reinterpret6/1
  data3/1 -> Assert3/1
  valid2/1 -> Logical10/3, Reinterpret4/1
  data2/1 -> Assert2/1
  valid1/1 -> Logical10/2, Reinterpret2/1
  data1/1 -> Assert1/1
  Assert7/1 -> Reinterpret15/1
  Reinterpret15/1 -> Logical7/1
  Convert7/1 -> Logical7/2
  Reinterpret14/1 -> Convert7/1
  Assert6/1 -> Reinterpret13/1
  Reinterpret13/1 -> Logical6/1
  Convert6/1 -> Logical6/2
  Reinterpret12/1 -> Convert6/1
  Assert5/1 -> Reinterpret11/1
  Reinterpret11/1 -> Logical5/1
  Convert5/1 -> Logical5/2
  Reinterpret10/1 -> Convert5/1
  Assert4/1 -> Reinterpret9/1
  Reinterpret9/1 -> Logical4/1
  Convert4/1 -> Logical4/2
  Reinterpret8/1 -> Convert4/1
  Assert3/1 -> Reinterpret7/1
  Reinterpret7/1 -> Logical3/1
  Convert3/1 -> Logical3/2
  Reinterpret6/1 -> Convert3/1
  Assert2/1 -> Reinterpret5/1
  Reinterpret5/1 -> Logical2/1
  Convert2/1 -> Logical2/2
  Reinterpret4/1 -> Convert2/1
  Assert1/1 -> Reinterpret3/1
  Reinterpret3/1 -> Logical1/1
  Convert1/1 -> Logical1/2
  Reinterpret2/1 -> Convert1/1
  Assert0/1 -> Reinterpret1/1
  Reinterpret1/1 -> Logical0/1
  Convert0/1 -> Logical0/2
  Reinterpret0/1 -> Convert0/1
  valid0/1 -> Logical10/1, Reinterpret0/1
  data0/1 -> Assert0/1

== system isi_correlator_lib/simple_bram_vacc/delay_bram ==
  In1 : Inport  OutDataType=sfix(16)  OutScaling=2^0
  Constant2 : xbsIndex_r4/Constant  arith_type=Boolean  const=1  n_bits=1  bin_pt=0  explicit_period=on  period=1  equ=P=C  opselect=C  inp2=PCIN>>17  opr=+  inp1=P  carry=CIN  dbl_ovrd=off  block_type=constant
  Counter : xbsIndex_r4/Counter  cnt_type=Count Limited  cnt_to=DelayLen - bram_latency - 1  operation=Up  start_count=0  cnt_by_val=1  arith_type=Unsigned  n_bits=BitWidth  bin_pt=0  load_pin=off  rst=off  en=off  explicit_period=off  period=1  dbl_ovrd=off  use_behavioral_HDL=off  implementation=Fabric  use_rpm=off  block_type=counter
      settings: xl_area=[0, 0, 0, 0, 0, 0, 0]
  Single Port RAM : xbsIndex_r4/Single Port RAM  depth=2^BitWidth  initVector=0  distributed_mem=Block RAM  write_mode=Read Before Write  rst=off  init_reg=0  en=off  latency=bram_latency  dbl_ovrd=off  optimize=Area  use_rpm=off  block_type=spram
      settings: xl_area=[0, 0, 0, 0, 0, 0, 0]  block_version=10.1.3
  Out1 : Outport  OutDataType=sfix(16)  OutScaling=2^0
  wires:
  Constant2/1 -> Single Port RAM/3
  In1/1 -> Single Port RAM/2
  Counter/1 -> Single Port RAM/1
  Single Port RAM/1 -> Out1/1

== system isi_correlator_lib/simple_bram_vacc/pulse_ext ==
  in : Inport  OutDataType=sfix(16)  OutScaling=2^0
  Constant5 : xbsIndex_r4/Constant  arith_type=Unsigned  const=pulse_len  n_bits=bits  bin_pt=0  explicit_period=off  period=1  equ=P=C  opselect=C  inp2=PCIN>>17  opr=+  inp1=P  carry=CIN  dbl_ovrd=off  block_type=constant
  Counter3 : xbsIndex_r4/Counter  cnt_type=Free Running  cnt_to=1023  operation=Up  start_count=0  cnt_by_val=1  arith_type=Unsigned  n_bits=bits  bin_pt=0  load_pin=off  rst=on  en=on  explicit_period=on  period=1  dbl_ovrd=off  use_behavioral_HDL=off  implementation=Fabric  use_rpm=on  block_type=counter
      settings: xl_area=[0, 0, 0, 0, 0, 0, 0]
  Relational5 : xbsIndex_r4/Relational  mode=a!=b  en=off  latency=0  dbl_ovrd=off  block_type=relational
      settings: xl_area=[0, 0, 0, 0, 0, 0, 0]  block_version=10.1.3
  posedge : Subsystem  Tag=Rising Edge Detector
  out : Outport  OutDataType=sfix(16)  OutScaling=2^0
  wires:
  Counter3/1 -> Relational5/1
  Constant5/1 -> Relational5/2
  Relational5/1 -> Counter3/2, out/1
  in/1 -> posedge/1(In)
  posedge/1(Out) -> Counter3/1

== system isi_correlator_lib/vacc/addr_counter ==
  en : Inport
  rst : Inport  Port=2
  Concat : xbsIndex_r4/Concat  num_inputs=2  dbl_ovrd=off  block_type=concat
  Constant3 : xbsIndex_r4/Constant  arith_type=Unsigned  const=72*5 - 1  n_bits=9  bin_pt=0  explicit_period=on  period=1  equ=P=C  opselect=C  inp2=PCIN>>17  opr=+  inp1=P  carry=CIN  dbl_ovrd=off  block_type=constant
      settings: block_version=11.4
  Constant4 : xbsIndex_r4/Constant  arith_type=Unsigned  const=0  n_bits=9  bin_pt=0  explicit_period=on  period=1  equ=P=C  opselect=C  inp2=PCIN>>17  opr=+  inp1=P  carry=CIN  dbl_ovrd=off  block_type=constant
      settings: block_version=11.4
  Inverter : xbsIndex_r4/Inverter  en=off  latency=0  dbl_ovrd=off  block_type=inv
      settings: block_version=11.3
  Logical1 : xbsIndex_r4/Logical  logical_function=AND  inputs=2  en=off  latency=0  precision=Full  arith_type=Unsigned  n_bits=16  bin_pt=0  align_bp=on  dbl_ovrd=off  block_type=logical
      settings: block_version=11.3
  Logical2 : xbsIndex_r4/Logical  logical_function=OR  inputs=2  en=off  latency=0  precision=Full  arith_type=Unsigned  n_bits=16  bin_pt=0  align_bp=on  dbl_ovrd=off  block_type=logical
      settings: block_version=11.3
  Logical3 : xbsIndex_r4/Logical  logical_function=OR  inputs=2  en=off  latency=0  precision=Full  arith_type=Unsigned  n_bits=16  bin_pt=0  align_bp=on  dbl_ovrd=off  block_type=logical
      settings: block_version=11.3
  Relational2 : xbsIndex_r4/Relational  mode=a=b  en=off  latency=0  dbl_ovrd=off  block_type=relational
  bram_addr : xbsIndex_r4/Counter  cnt_type=Free Running  cnt_to=Inf  operation=Up  start_count=0  cnt_by_val=1  arith_type=Unsigned  n_bits=9  bin_pt=0  load_pin=on  rst=off  en=on  explicit_period=on  period=1  dbl_ovrd=off  use_behavioral_HDL=off  implementation=Fabric  use_rpm=off  block_type=counter
  bram_slot : xbsIndex_r4/Counter  cnt_type=Free Running  cnt_to=Inf  operation=Up  start_count=0  cnt_by_val=1  arith_type=Unsigned  n_bits=1  bin_pt=0  load_pin=off  rst=on  en=on  explicit_period=on  period=1  dbl_ovrd=off  use_behavioral_HDL=off  implementation=Fabric  use_rpm=off  block_type=counter
  packet_id : xbsIndex_r4/Counter  cnt_type=Free Running  cnt_to=Inf  operation=Up  start_count=0  cnt_by_val=1  arith_type=Unsigned  n_bits=22  bin_pt=0  load_pin=off  rst=on  en=on  explicit_period=on  period=1  dbl_ovrd=off  use_behavioral_HDL=off  implementation=Fabric  use_rpm=off  block_type=counter
  rst_filter : Subsystem
  pkt_id : Outport
  addr : Outport  Port=2
  we : Outport  Port=3
  wires:
  Logical2/1 -> bram_addr/1, Logical3/1
  Constant4/1 -> bram_addr/2
  Logical3/1 -> bram_addr/3
  en/1 -> rst_filter/1(en)
  rst/1 -> rst_filter/2(rst)
  bram_addr/1 -> Concat/2, Relational2/2
  Constant3/1 -> Relational2/1
  Logical1/1 -> we/1
  Relational2/1 -> Logical2/1, packet_id/2, bram_slot/2
  Inverter/1 -> Logical1/2
  rst_filter/2(r) -> Inverter/1, bram_slot/1, packet_id/1, Logical2/2
  rst_filter/1(e) -> Logical3/2, Logical1/1
  bram_slot/1 -> Concat/1
  Concat/1 -> addr/1
  packet_id/1 -> pkt_id/1

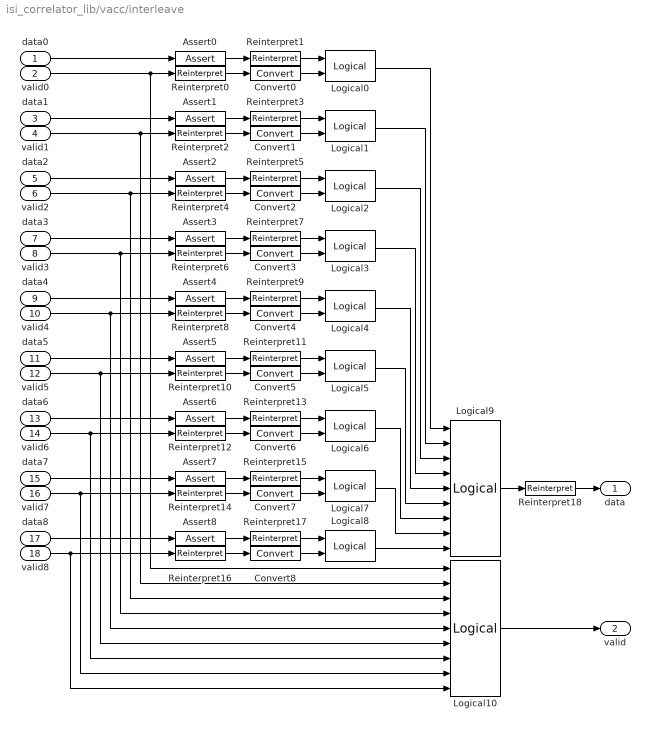
== system isi_correlator_lib/vacc/interleave ==
  data0 : Inport
  valid0 : Inport  Port=2
  data1 : Inport  Port=3
  valid1 : Inport  Port=4
  data2 : Inport  Port=5
  valid2 : Inport  Port=6
  data3 : Inport  Port=7
  valid3 : Inport  Port=8
  data4 : Inport  Port=9
  valid4 : Inport  Port=10
  data5 : Inport  Port=11
  valid5 : Inport  Port=12
  data6 : Inport  Port=13
  valid6 : Inport  Port=14
  data7 : Inport  Port=15
  valid7 : Inport  Port=16
  data8 : Inport  Port=17
  valid8 : Inport  Port=18
  Assert{0..8} (9 alike) : xbsIndex_r4/Assert  assert_type=on  type_source=Explicitly  arith_type="Signed  (2's comp)"  n_bits=bit_width  bin_pt=bin_point  assert_rate=on  rate_source=Explicitly  period=1  output_port=on  block_type=assert
      settings: block_version=11.4
  Convert{0..8} (9 alike) : xbsIndex_r4/Convert  arith_type="Signed  (2's comp)"  n_bits=bit_width  bin_pt=0  quantization=Truncate  overflow=Wrap  latency=0  dbl_ovrd=off  pipeline=off  block_type=convert
      settings: block_version=11.4
  Logical{0..8} (9 alike) : xbsIndex_r4/Logical  logical_function=AND  inputs=2  en=off  latency=logic_latency  precision=Full  arith_type=Unsigned  n_bits=16  bin_pt=0  align_bp=on  dbl_ovrd=off  block_type=logical
      settings: block_version=11.3
  Logical10 : xbsIndex_r4/Logical  logical_function=OR  inputs=9  en=off  latency=logic_latency + fanin_latency  precision=Full  arith_type=Unsigned  n_bits=16  bin_pt=0  align_bp=on  dbl_ovrd=off  block_type=logical
      settings: block_version=11.3
  Logical9 : xbsIndex_r4/Logical  logical_function=OR  inputs=9  en=off  latency=fanin_latency  precision=Full  arith_type=Unsigned  n_bits=16  bin_pt=0  align_bp=on  dbl_ovrd=off  block_type=logical
      settings: block_version=11.3
  Reinterpret{0,2,4,6,8,10,12,14,16} (9 alike) : xbsIndex_r4/Reinterpret  force_arith_type=on  arith_type="Signed  (2's comp)"  force_bin_pt=on  bin_pt=0  block_type=reinterpret
      settings: infoedit="Changes signal type without altering the binary representation.   You can changed the signal between signed and unsigned, and relocate the binary point.<br><br>Hardware notes: In hardware this block costs nothing.<br><br>Example:  Suppose the input is 6 bits wide, signed, with 2 fractional bits, and the output is forced to unsigned with 0 fractional bits.  Then an input of -2.0 (1110.00 in binary 2's complement) becomes an output of 56 (111000 in binary)."
  Reinterpret{1,3,5,7,9,11,13,15,17} (9 alike) : xbsIndex_r4/Reinterpret  force_arith_type=on  arith_type=Unsigned  force_bin_pt=on  bin_pt=0  block_type=reinterpret
      settings: infoedit="Changes signal type without altering the binary representation.   You can changed the signal between signed and unsigned, and relocate the binary point.<br><br>Hardware notes: In hardware this block costs nothing.<br><br>Example:  Suppose the input is 6 bits wide, signed, with 2 fractional bits, and the output is forced to unsigned with 0 fractional bits.  Then an input of -2.0 (1110.00 in binary 2's complement) becomes an output of 56 (111000 in binary)."
  Reinterpret18 : xbsIndex_r4/Reinterpret  force_arith_type=on  arith_type="Signed  (2's comp)"  force_bin_pt=on  bin_pt=bin_point  block_type=reinterpret
      settings: infoedit="Changes signal type without altering the binary representation.   You can changed the signal between signed and unsigned, and relocate the binary point.<br><br>Hardware notes: In hardware this block costs nothing.<br><br>Example:  Suppose the input is 6 bits wide, signed, with 2 fractional bits, and the output is forced to unsigned with 0 fractional bits.  Then an input of -2.0 (1110.00 in binary 2's complement) becomes an output of 56 (111000 in binary)."
  data : Outport
  valid : Outport  Port=2
  wires:
  data0/1 -> Assert0/1
  valid0/1 -> Reinterpret0/1, Logical10/1
  Reinterpret0/1 -> Convert0/1
  Convert0/1 -> Logical0/2
  Reinterpret1/1 -> Logical0/1
  Assert0/1 -> Reinterpret1/1
  Reinterpret2/1 -> Convert1/1
  Convert1/1 -> Logical1/2
  Reinterpret3/1 -> Logical1/1
  Assert1/1 -> Reinterpret3/1
  Reinterpret4/1 -> Convert2/1
  Convert2/1 -> Logical2/2
  Reinterpret5/1 -> Logical2/1
  Assert2/1 -> Reinterpret5/1
  Reinterpret6/1 -> Convert3/1
  Convert3/1 -> Logical3/2
  Reinterpret7/1 -> Logical3/1
  Assert3/1 -> Reinterpret7/1
  Reinterpret8/1 -> Convert4/1
  Convert4/1 -> Logical4/2
  Reinterpret9/1 -> Logical4/1
  Assert4/1 -> Reinterpret9/1
  Reinterpret10/1 -> Convert5/1
  Convert5/1 -> Logical5/2
  Reinterpret11/1 -> Logical5/1
  Assert5/1 -> Reinterpret11/1
  Reinterpret12/1 -> Convert6/1
  Convert6/1 -> Logical6/2
  Reinterpret13/1 -> Logical6/1
  Assert6/1 -> Reinterpret13/1
  Reinterpret14/1 -> Convert7/1
  Convert7/1 -> Logical7/2
  Reinterpret15/1 -> Logical7/1
  Assert7/1 -> Reinterpret15/1
  Reinterpret16/1 -> Convert8/1
  Convert8/1 -> Logical8/2
  Reinterpret17/1 -> Logical8/1
  Assert8/1 -> Reinterpret17/1
  data1/1 -> Assert1/1
  valid1/1 -> Reinterpret2/1, Logical10/2
  data2/1 -> Assert2/1
  valid2/1 -> Reinterpret4/1, Logical10/3
  data3/1 -> Assert3/1
  valid3/1 -> Reinterpret6/1, Logical10/4
  data4/1 -> Assert4/1
  valid4/1 -> Reinterpret8/1, Logical10/5
  data5/1 -> Assert5/1
  valid5/1 -> Reinterpret10/1, Logical10/6
  data6/1 -> Assert6/1
  valid6/1 -> Reinterpret12/1, Logical10/7
  data7/1 -> Assert7/1
  valid7/1 -> Reinterpret14/1, Logical10/8
  data8/1 -> Assert8/1
  valid8/1 -> Reinterpret16/1, Logical10/9
  Logical8/1 -> Logical9/9
  Logical9/1 -> Reinterpret18/1
  Reinterpret18/1 -> data/1
  Logical10/1 -> valid/1
  Logical0/1 -> Logical9/1
  Logical1/1 -> Logical9/2
  Logical2/1 -> Logical9/3
  Logical3/1 -> Logical9/4
  Logical4/1 -> Logical9/5
  Logical5/1 -> Logical9/6
  Logical6/1 -> Logical9/7
  Logical7/1 -> Logical9/8

== system isi_correlator_lib/packed_bram/addr_counter/rst_filter ==
  en : Inport
  rst : Inport  Port=2
  Delay : xbsIndex_r4/Delay  en=off  latency=1  dbl_ovrd=off  reg_retiming=off  block_type=delay
      settings: xl_area=[0, 0, 0, 0, 0, 0, 0]  block_version=9.1.01
  Delay1 : xbsIndex_r4/Delay  en=off  latency=1  dbl_ovrd=off  reg_retiming=off  block_type=delay
      settings: xl_area=[0, 0, 0, 0, 0, 0, 0]  block_version=9.1.01
  Inverter1 : xbsIndex_r4/Inverter  en=off  latency=0  dbl_ovrd=off  block_type=inv
      settings: block_version=11.3
  Inverter2 : xbsIndex_r4/Inverter  en=off  latency=0  dbl_ovrd=off  block_type=inv
      settings: block_version=11.3
  Inverter3 : xbsIndex_r4/Inverter  en=off  latency=0  dbl_ovrd=off  block_type=inv
      settings: block_version=11.3
  Logical1 : xbsIndex_r4/Logical  logical_function=AND  inputs=2  en=off  latency=0  precision=Full  arith_type=Unsigned  n_bits=16  bin_pt=0  align_bp=on  dbl_ovrd=off  block_type=logical
      settings: block_version=11.3
  Logical2 : xbsIndex_r4/Logical  logical_function=AND  inputs=2  en=off  latency=0  precision=Full  arith_type=Unsigned  n_bits=16  bin_pt=0  align_bp=on  dbl_ovrd=off  block_type=logical
      settings: block_version=11.3
  Logical3 : xbsIndex_r4/Logical  logical_function=OR  inputs=2  en=off  latency=0  precision=Full  arith_type=Unsigned  n_bits=16  bin_pt=0  align_bp=on  dbl_ovrd=off  block_type=logical
      settings: block_version=11.3
  Logical4 : xbsIndex_r4/Logical  logical_function=AND  inputs=2  en=off  latency=0  precision=Full  arith_type=Unsigned  n_bits=16  bin_pt=0  align_bp=on  dbl_ovrd=off  block_type=logical
      settings: block_version=11.3
  Register : xbsIndex_r4/Register  init=0  rst=on  en=on  dbl_ovrd=off  block_type=register
      settings: block_version=11.4
  e : Outport
  r : Outport  Port=2
  wires:
  Logical1/1 -> Register/1, Register/3
  Inverter1/1 -> Logical2/1
  Inverter2/1 -> Logical2/2
  Register/1 -> Logical3/1, Inverter3/1
  Logical3/1 -> r/1
  rst/1 -> Logical1/2, Inverter2/1, Delay1/1
  en/1 -> Delay/1, Inverter1/1, Logical1/1
  Logical2/1 -> Register/2
  Logical4/1 -> e/1
  Delay/1 -> Logical4/1
  Inverter3/1 -> Logical4/2
  Delay1/1 -> Logical3/2

== system isi_correlator_lib/simple_bram_vacc/pulse_ext/posedge ==
  In : Inport  OutDataType=sfix(16)  OutScaling=2^0
  Delay : xbsIndex_r4/Delay  en=off  latency=1  dbl_ovrd=off  reg_retiming=off  block_type=delay
      settings: xl_area=[0, 0, 0, 0, 0, 0, 0]
  Inverter : xbsIndex_r4/Inverter  en=off  latency=0  dbl_ovrd=off  block_type=inv
      settings: xl_area=[0, 0, 0, 0, 0, 0, 0]
  Logical : xbsIndex_r4/Logical  logical_function=AND  inputs=2  en=off  latency=0  precision=Full  arith_type=Unsigned  n_bits=8  bin_pt=2  align_bp=on  dbl_ovrd=off  block_type=logical
      settings: xl_area=[0, 0, 0, 0, 0, 0, 0]
  Out : Outport  OutDataType=sfix(16)  OutScaling=2^0
  wires:
  Delay/1 -> Inverter/1
  Inverter/1 -> Logical/1
  In/1 -> Delay/1, Logical/2
  Logical/1 -> Out/1
